simulink model "W01_interactive"  (R2024b)
settings: Solver=ode4  StartTime=0  StopTime=inf  FixedStep=h  RelTol=1e-3
PostLoadFcn:
  | p_ = fileparts(get_param(bdroot,'FileName')); addpath(p_, fullfile(fileparts(fileparts(p_)),'_tools')); mss_path(); clear p_
StartFcn:
  | if isappdata(0,'W01i_n'), rmappdata(0,'W01i_n'); end
model workspace (MAT data in the model file):
  V_c = 0
  animate = 1
  beta_c = 0
  h = 0.02
  mp = 25
  rp = [0.05; 0; -0.35]
  x0 = [0; 0; 0; 0; 0; 0; 0; 0; 0; 0; 0; 0]
settings Model: Creator=admin  LastModifiedBy=admin
settings DataIOCC: ReturnWorkspaceOutputs=off

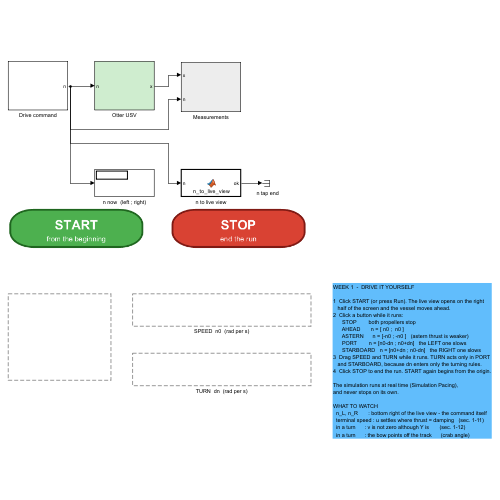
[thumbnail: Simulink's stored preview of the top-level diagram]
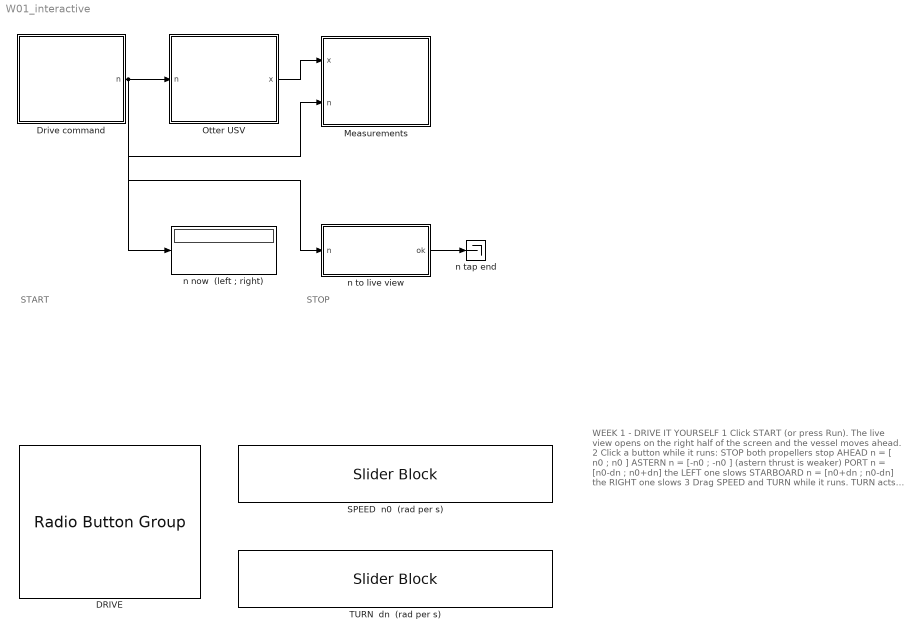
== system W01_interactive ==
  note: START
  note: STOP
  note: WEEK 1  -  DRIVE IT YOURSELF
      |
      | 1  Click START (or press Run). The live view opens on the right
      |    half of the screen and the vessel moves ahead.
      | 2  Click a button while it runs:
      |       STOP        both propellers stop
      |       AHEAD       n = [ n0 ;  n0 ]
      |       ASTERN      n = [-n0 ; -n0 ]   (astern thrust is weaker)
      |       PORT        n = [n0-dn ; n0+dn]   the LEFT one slows
      |       STARBOARD   n = [n0+dn ; n0-dn]   the RIGHT one slows
      | 3  Drag SPEED and TURN while it runs. TURN acts only in PORT
      |    and STARBOARD, because dn enters only the turning rules.
      | 4  Click STOP to end the run. START again begins from the origin.
      |
      | The simulation runs at real time (Simulation Pacing),
      | and never stops on its own.
      |
      | WHAT TO WATCH
      |   n_L, n_R       : bottom right of the live view - the command itself
      |   terminal speed : u settles where thrust = damping   (sec. 1-11)
      |   in a turn      : v is not zero although Y is       (sec. 1-12)
      |   in a turn      : the bow points off the track      (crab angle)
  DRIVE : RadioButtonGroup  SelectedLabel=AHEAD  ButtonGroupName=DRIVE
      settings: Values={{'STOP', 'AHEAD', 'ASTERN', 'PORT (left)', 'STARBOARD (right)'}, [0 1 2 3 4]}
  Drive command : Subsystem
  Measurements : Subsystem
  Otter USV : Subsystem
  SPEED  n0  (rad per s) : SliderBlock
  TURN  dn  (rad per s) : SliderBlock  ScaleMax=30
  n now  (left ; right) : Display
  n tap end : Terminator
  n to live view : MATLAB Function  TreatAsAtomicUnit=on
  wires:
  Drive command/1(n) -> Otter USV/1(n), Measurements/2(n), n now  (left ; right)/1, n to live view/1(n)
  Otter USV/1(x) -> Measurements/1(x)
  n to live view/1(ok) -> n tap end/1

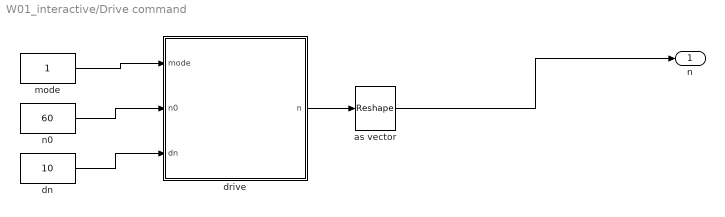
== system W01_interactive/Drive command ==
  as vector : Reshape
  dn : Constant  Value=10
  drive : MATLAB Function  TreatAsAtomicUnit=on
  mode : Constant
  n0 : Constant  Value=60
  n : Outport
  wires:
  mode/1 -> drive/1(mode)
  n0/1 -> drive/2(n0)
  dn/1 -> drive/3(dn)
  drive/1(n) -> as vector/1
  as vector/1 -> n/1

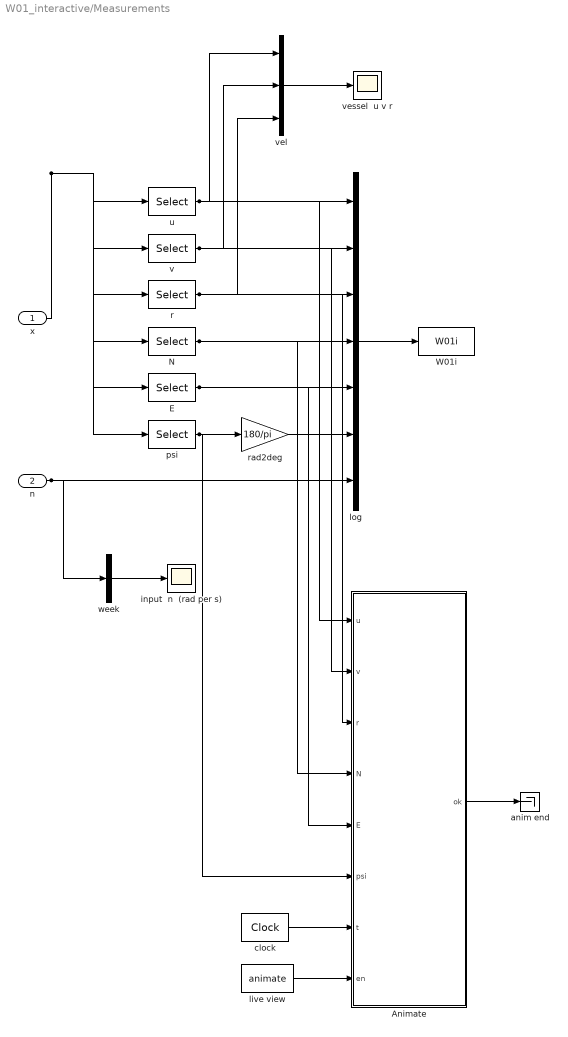
== system W01_interactive/Measurements ==
  x : Inport
  n : Inport  Port=2
  Animate : MATLAB Function  TreatAsAtomicUnit=on
  E : Selector  InputPortWidth=12  IndexOptions=Index vector (dialog)  Indices=8  OutputSizes=1
  N : Selector  InputPortWidth=12  IndexOptions=Index vector (dialog)  Indices=7  OutputSizes=1
  W01i : ToWorkspace  VariableName=W01i  SaveFormat=Structure With Time  SampleTime=-1
  anim end : Terminator
  clock : DigitalClock  SampleTime=h
  input  n  (rad per s) : Scope
  live view : Constant  Value=animate
  log : Mux  Inputs=7
  psi : Selector  InputPortWidth=12  IndexOptions=Index vector (dialog)  Indices=12  OutputSizes=1
  r : Selector  InputPortWidth=12  IndexOptions=Index vector (dialog)  Indices=6  OutputSizes=1
  rad2deg : Gain  Gain=180/pi
  u : Selector  InputPortWidth=12  IndexOptions=Index vector (dialog)  Indices=1  OutputSizes=1
  v : Selector  InputPortWidth=12  IndexOptions=Index vector (dialog)  Indices=2  OutputSizes=1
  vel : Mux  Inputs=3
  vessel  u v r : Scope
  week : Mux  Inputs=1
  wires:
  x/1 -> u/1, v/1, r/1, N/1, E/1, psi/1
  log/1 -> W01i/1
  psi/1 -> rad2deg/1, Animate/6(psi)
  u/1 -> log/1, vel/1, Animate/1(u)
  v/1 -> log/2, vel/2, Animate/2(v)
  r/1 -> log/3, vel/3, Animate/3(r)
  N/1 -> log/4, Animate/4(N)
  E/1 -> log/5, Animate/5(E)
  rad2deg/1 -> log/6
  n/1 -> log/7, week/1
  vel/1 -> vessel  u v r/1
  week/1 -> input  n  (rad per s)/1
  clock/1 -> Animate/7(t)
  live view/1 -> Animate/8(en)
  Animate/1(ok) -> anim end/1

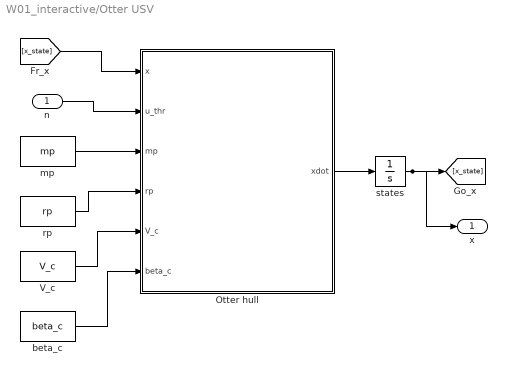
== system W01_interactive/Otter USV ==
  n : Inport
  Otter hull : MATLAB Function  TreatAsAtomicUnit=on
  V_c : Constant  Value=V_c
  beta_c : Constant  Value=beta_c
  mp : Constant  Value=mp
  rp : Constant  Value=rp
  states : Integrator  InitialCondition=x0
  x : Outport
  wires:
  V_c/1 -> Otter hull/5(V_c)
  [x_state] -> Otter hull/1(x)
  mp/1 -> Otter hull/3(mp)
  n/1 -> Otter hull/2(u_thr)
  rp/1 -> Otter hull/4(rp)
  beta_c/1 -> Otter hull/6(beta_c)
  Otter hull/1(xdot) -> states/1
  states/1 -> [x_state], x/1

== matlab function W01_interactive/Otter USV/Otter hull ==
  data: x input; xdot output double size=[12 1]; u_thr input; mp input; rp input; V_c input; beta_c input
function xdot = otter_hull(x, u_thr, mp, rp, V_c, beta_c)
% Fossen's otter.m, called unchanged from Tools/MSS/VESSELS.
%
%   x       12 states, fed back from the integrator
%   u_thr   propeller shaft speeds [rad/s]
%
% otter.m is not written for code generation, so the call is extrinsic and
% xdot has to be pre-sized for Simulink to know the output width.
coder.extrinsic('otter');

xdot = zeros(12,1);
xdot = otter(x, u_thr, mp, rp, V_c, beta_c);
end

== matlab function W01_interactive/Drive command/drive ==
  data: mode input; n output double size=[2 1]; n0 input; dn input
function n = drive(mode, n0, dn)
%#codegen
%DRIVE  Turn one button into two shaft speeds.
%
%   mode   0 STOP, 1 AHEAD, 2 ASTERN, 3 PORT, 4 STARBOARD   (the buttons)
%   n0     common shaft speed [rad/s]                         (SPEED slider)
%   dn     difference between the two in a turn [rad/s]       (TURN slider)
%
%   The yaw moment is N = y_p (T_left - T_right), so a PORT turn slows
%   the LEFT propeller - the same rule as the timetable of W01_openloop.

switch mode
    case 1,    n = [ n0;       n0      ];   % AHEAD
    case 2,    n = [-n0;      -n0      ];   % ASTERN
    case 3,    n = [ n0 - dn;  n0 + dn ];   % PORT
    case 4,    n = [ n0 + dn;  n0 - dn ];   % STARBOARD
    otherwise, n = [ 0;        0       ];   % STOP
end

== matlab function W01_interactive/Measurements/Animate ==
  data: u input; ok output; v input; r input; N input; E input; psi input; t input; en input
function ok = Animate(u, v, r, N, E, psi, t, en)
%#codegen
% Live view of the vessel while the model runs.
%
% A MATLAB Function block cannot plot, so the drawing function is declared
% extrinsic: Simulink calls plain MATLAB rather than generating code for it.
% Set animate = 0 in the setup script to switch the live view off.
%
% psi arrives in RADIANS and r in rad/s - the units otter.m works in. The
% wrapper converts them for display, in one place, so no two figures in the
% course can disagree about what a degree is.
coder.extrinsic('W01i_animate');
ok = 1;
if en > 0.5
    W01i_animate(u, v, r, N, E, psi, t);
end
end

== matlab function W01_interactive/n to live view ==
  data: n input; ok output double size=1
function ok = n_to_live_view(n)
%#codegen
%N_TO_LIVE_VIEW  Hand the two shaft speeds to the live view.
%
%   The Animate block inside Measurements receives only the vessel states.
%   W01i_animate reads the latest n from here and plots n_L and n_R.
coder.extrinsic('setappdata');
setappdata(0, 'W01i_n', n);
ok = 1;
